simulink model "zynqRadioHWSWQPSKAD9361AD9364SL"  (R2025a)
settings: Solver=FixedStepDiscrete  StartTime=0.0  StopTime=0.5  RelTol=1e-3
PreLoadFcn:
  | setTxBurstLength = 10000;
  | txtmsg = ['Zynq radio HW/SW Co-design ÞÞÞÞ']; % Use only printable characters
  | 
  | %------------------------------------------------------------------------------------------------------
  | if ~isequal(size(txtmsg),[1 31])
  |     error('txtmsg must contain 31 characters');
  | end
  | 
  | [dataBits,msg] = zynqRadioHWSWQPSKgenHelloworldMsg(20); % generate 20 msgs for LUT
  | msgLUT = uint8(msg);
  | dataBitsLUT = dataBits(:);
  | Rsym                = 10e3;%1.92e6;
  | Config = zynqRadioHWSWQPSKTxRxParameters;
  | fs = Rsym*Config.SamplesPerSymbol;
  | word = [txtmsg newline];  % append a new line character to txtmsg
  | 
  | % The highest clock rate is 16 times the message character rate.
  | % As the message characters are fed at highest clock to FPGA
  | % repeat each character 16 times to maintain the message rate.
  | word = repelem(word.',16,1);
  | repeatTimes = ceil(setTxBurstLength/length(word));
  | inpData = complex(repmat(uint8(word),repeatTimes,1));
  | inUseTxBurstLength = length(inpData);
PostLoadFcn:
  | hScopeConfig = get_param([gcs '/HDL_QPSK/QPSK Tx Channel QPSK Rx/QPSK Rx/Frequency and Time Synchronizer/Symbol Synchronizer/No HDL/QPSK Receiver Eye Diagram'],'ScopeConfiguration');
  | hScopeConfig.OpenAtSimulationStart = false;
  | hScopeConfig.Visible = false;
  | clear hScopeConfig
InitFcn:
  | setTxBurstLength = 10000;
  | txtmsg = ['Zynq radio HW/SW Co-design ÞÞÞÞ']; % Use only printable characters
  | 
  | %------------------------------------------------------------------------------------------------------
  | if ~isequal(size(txtmsg),[1 31])
  |     error('txtmsg must contain 31 characters');
  | end
  | 
  | [dataBits,msg] = zynqRadioHWSWQPSKgenHelloworldMsg(20); % generate 20 msgs for LUT
  | msgLUT = uint8(msg);
  | dataBitsLUT = dataBits(:);
  | Rsym                = 10e3;%1.92e6;
  | Config = zynqRadioHWSWQPSKTxRxParameters;
  | fs = Rsym*Config.SamplesPerSymbol;
  | word = [txtmsg newline];  % append a new line character to txtmsg
  | 
  | % The highest clock rate is 16 times the message character rate.
  | % As the message characters are fed at highest clock to FPGA
  | % repeat each character 16 times to maintain the message rate.
  | word = repelem(word.',16,1);
  | repeatTimes = ceil(setTxBurstLength/length(word));
  | inpData = complex(repmat(uint8(word),repeatTimes,1));
  | inUseTxBurstLength = length(inpData);
  | 
  | Config.Preamble = logical(zeros(0,1))
undefined symbols (not defined in the file or in its folder): Add, dspblkCoreblockFVToolHelper, gcbh, gse_genframes, Shift
libraries: hdlsllib x144, simulink x37, dsphdlsigops2 x3, dsphdlfiltering2 x3, whdlutilities x3, dsphdlxfrm2 x2, dsphdlmathfun2 x2, commdigbbndpm3 x2, sdrzblksprivate x1
(part 6 of 6)

== matlab function zynqRadioHWSWQPSKAD9361AD9364SL/HDL_QPSK/QPSK Tx Channel QPSK Rx/QPSK Tx/FEC Encoder/DVB-S2 LDPC Encoder/ParityController ==
  data: ird_addr output; pwr_addr output; pwr_enb output; prd_addr output; endEnc input; paraddr input; encenable input; inpLen input; parLen input; qfactor input; noofcol input; reset input; starto output; endo output; valido output; par_ind output; i_index output; p_index output; framevalid input
function [ird_addr,pwr_addr,pwr_enb,prd_addr,starto,endo,valido,par_ind,...
    i_index,p_index] = ParityController(endEnc,paraddr,encenable,...
    inpLen,parLen,qfactor,noofcol,reset,framevalid)

persistent validO prdAddr pwrAddr pwrEnb pwrEnbReg ...
    irdAddr prdEnb endValid startO icountZ inCount ...
    parCount pcountZ outCount;
if isempty(validO)
    validO = false;
    prdAddr = uint8(1);
    pwrAddr = uint8(0);
    irdAddr = uint8(1);
    pwrEnb = false;
    pwrEnbReg = false;
    prdEnb = false;
    endValid = false;
    startO = false;
    icountZ = fi(1,0,9,0,hdlfimath);
    pcountZ = fi(1,0,9,0,hdlfimath);
    inCount = fi(0,0,16,0,hdlfimath);
    parCount = fi(0,0,16,0,hdlfimath);
    outCount = fi(0,0,16,0,hdlfimath);
end

ird_addr = irdAddr;
pwr_addr = pwrAddr;
prd_addr = prdAddr;
pwr_enb =  pwrEnbReg;
starto = startO;
par_ind = prdEnb;

i_index = icountZ;
p_index = pcountZ;

% Control signals
startO = endEnc;
endo = endValid;
valido = validO;

pwrEnbReg(:) = pwrEnb;

if reset
    prdAddr(:) = 1;
    pwrAddr(:) = 0;
    pwrEnb(:) = false;
    prdEnb(:) = false;
    irdAddr(:) = 1;
    icountZ(:) = 1;
    pcountZ(:) = 1;
    inCount(:) = 0;
    parCount(:) = 0;
else
    if validO
        pwrEnb(:) = false;
        pwrAddr(:) = 0;

        if ~prdEnb
            if icountZ == fi(360,0,9,0,hdlfimath)
                if ~(irdAddr == noofcol)
                    irdAddr(:) = irdAddr + 1;
                end
                icountZ(:) = 1;
            else
                icountZ(:) = icountZ + 1;
            end
        end

        if inCount == inpLen
            prdEnb(:) = true;
        else
            inCount(:) = inCount + 1;
        end

        if prdEnb
            if parCount == parLen
                prdEnb(:) = false;
            else
                parCount(:) = parCount + 1;
                if prdAddr == fi(qfactor,0,9,0,hdlfimath)
                    prdAddr(:) = 1;
                    if pcountZ == fi(360,0,9,0,hdlfimath)
                        pcountZ(:) = 1;
                    else
                        pcountZ(:) = pcountZ + 1;
                    end
                else
                    prdAddr(:) = prdAddr + 1;
                end
            end
        else
            prdAddr(:) = 1;
        end
    else
        if framevalid
            pwrEnb(:) = true;
            if pwrAddr == uint8(255)
                pwrAddr(:) = 1;
            else
                pwrAddr(:) = pwrAddr+1;
            end
        else
            if encenable
                pwrEnb(:) = true;
            else
                pwrEnb(:) = false;
            end
            pwrAddr(:) = prdAddr;
        end
        prdAddr(:) = paraddr;
        prdEnb(:) = false;
    end
end

if reset
    validO(:) = false;
    outCount(:) = 0;
elseif endEnc
    validO(:) = true;
    outCount(:) = 1;
else
    if validO
        if outCount == inpLen + parLen
            endValid(:) = true;
            outCount(:) = 0;
            validO(:) = false;
        else
            endValid(:) = false;
            outCount(:) = outCount+1;
        end
    else
        validO(:) = false;
        endValid(:) = false;
    end
end

== matlab function zynqRadioHWSWQPSKAD9361AD9364SL/HDL_QPSK/QPSK Tx Channel QPSK Rx/QPSK Tx/FEC Encoder/DVB-S2 LDPC Encoder/inputController ==
  data: reset output; datai input; iwr_data output size=360; iwr_addr output; starti input; endi input; validi input; fecframe input; coderate input; iwr_enb output size=1; ird_addr output; encenable output; addridx output; rdenable input; encend input; framevalid output; noofcol input
function [reset,iwr_data, iwr_addr,iwr_enb,ird_addr,encenable,addridx,framevalid] = ...
    inputController(datai,starti,endi,validi,fecframe,coderate,rdenable,encend,noofcol)
%#codegen

persistent fecFrame codeRate dataReg endReg validReg frameValid  frameValidReg...
           iwrData iwrAddr iwrEnb irdAddr idxCount wrCount encEnb disValid;
if isempty(dataReg)
    fecFrame = fi(0,0,1,0);
    codeRate = fi(0,0,4,0);
    dataReg = cast(0,'like',datai);
    endReg = false;
    validReg = false;
    frameValid = false;
    frameValidReg = false;
    iwrData = cast(zeros(360,1),'like',datai);
    iwrAddr = fi(0,0,8,0,hdlfimath);
    iwrEnb  = zeros(1,1)>0;
    irdAddr = fi(0,0,8,0,hdlfimath);
    idxCount = fi(1,0,9,0,hdlfimath);
    wrCount = fi(1,0,8,0,hdlfimath);
    encEnb = false;
    disValid = false;
end

% outputs
iwr_data = iwrData;
iwr_addr = iwrAddr;
iwr_enb = iwrEnb;
ird_addr = irdAddr;
encenable = disValid;

%% reset signal
reset = starti && validi;

%% Sample fecFrame and codeRate - Calculate input,parity length and address index.
if reset
    fecFrame(:) = fecframe;
    codeRate(:) = coderate;
end

addridx = fi(bitconcat(fecFrame,codeRate),0,5,0);

%% Reading data
if reset
    irdAddr(:) = 1;
else
    if rdenable
        if irdAddr == cast(noofcol,'like',irdAddr)
            irdAddr(:) = 1;
        else
            irdAddr(:) = irdAddr + 1;
        end
    end
end

%% Writing and Reading data into Input Bits RAM
if reset
    iwrData(:) = zeros(360,1);
    iwrAddr(:) = 0;
    iwrEnb(:) = zeros(1,1);
    idxCount(:) = 1;
    wrCount(:) = 1;
else
    if frameValid && validReg
         iwrEnb = true;
        for idx = 1:360
            if idxCount == fi(idx,0,9,0)
                iwrData(idx) = dataReg;
            end
        end
        iwrAddr(:) = wrCount;
        if idxCount == fi(360,0,9,0)
            idxCount(:) = 1;
            wrCount(:) = wrCount + 1;
        else
            idxCount(:) = idxCount + 1;
        end
    else
        % iwrData(:) = 0;
        iwrEnb(:)  = false;
    end
end

if reset
    frameValid(:) = true;
    encEnb(:) = false;
elseif endReg && validReg
    frameValid(:) = false;
    encEnb(:) = true;
elseif encend
    encEnb(:) = false;
end

if reset
    frameValidReg(:) = true;
elseif endi && validi
    frameValidReg(:) = false;
end

if encEnb
    disValid(:) = ~disValid;
else
    disValid(:) = false;
end

framevalid = frameValidReg;

dataReg(:) = datai;
endReg(:) = endi;
validReg(:) = validi;

== matlab function zynqRadioHWSWQPSKAD9361AD9364SL/HDL_QPSK/QPSK Tx Channel QPSK Rx/QPSK Rx/Frequency and Time Synchronizer/Packet Controller/MATLAB Function ==
  data: valid input; syncPulse input; out output
function out = fcn(valid,syncPulse)
%#codegen

  persistent Reg;
  if isempty(Reg)
      Reg = false;
  end
  
  out = Reg;
  
  if Reg && valid
      Reg = false;
  end
  
  if syncPulse
      Reg = true;
  end
  
end

== matlab function zynqRadioHWSWQPSKAD9361AD9364SL/HDL_QPSK/QPSK Tx Channel QPSK Rx/QPSK Rx/Frequency and Time Synchronizer/Symbol Synchronizer/Rate Handle/FIFO/Validate Input Push Pop/MATLAB Function ==
  data: rst input; count output; enb input; dir input; initVal parameter; countToVal parameter
function count = hdlCounter(rst,enb,dir,initVal,countToVal)
%#codegen

persistent countReg

if(isempty(countReg))
    countReg = fi(initVal,0,nextpow2(countToVal+1),0);
end

if(rst)
    countReg(:) = initVal;
elseif(enb)
    if(dir)
        if(countReg==countToVal)
            countReg(:) = initVal;
        else
            countReg(:) = countReg+1;
        end
    else
        if(countReg==initVal)
            countReg(:) = countToVal;
        else
            countReg(:) = countReg-1;
        end
    end
end

count = countReg;

end

== matlab function zynqRadioHWSWQPSKAD9361AD9364SL/HDL_QPSK/QPSK Tx Channel QPSK Rx/QPSK Tx/Bit Packetizer/Data Bits FIFO/MATLAB Function1 ==
  data: wr input; full output; rd input; dataBitsPerPacket parameter
function full = fcn(wr,rd,dataBitsPerPacket)
%#codegen
     
    depth = dataBitsPerPacket*2 - 1;
    persistent count;
    if isempty(count)
        count = fi(0,0,nextpow2(depth),0,hdlfimath);
    end

    if wr
        count(:) = count + 1;
    end
    if rd
        count(:) = count - 1;
    end

    full = (count > depth);

end

== matlab function zynqRadioHWSWQPSKAD9361AD9364SL/HDL_QPSK/QPSK Tx Channel QPSK Rx/QPSK Rx/Frequency and Time Synchronizer/Packet Controller/sample discard controller ==
  data: dataIn input; validIn input; dataOut output; startIn input; endIn input; startOut output; endOut output; validOut output
function [dataOut,startOut,endOut,validOut] = controller(dataIn,validIn,startIn,endIn)
%#codegen

   persistent active dataOutReg validOutReg startOutReg endOutReg;
   if isempty(active)
      active  = false;
      dataOutReg = cast(0,'like',dataIn);
      validOutReg = false;
      startOutReg = false;
      endOutReg = false;
   end
   
   dataOut = dataOutReg;
   validOut = validOutReg;
   startOut = startOutReg;
   endOut = endOutReg;
   
   startOutReg = startIn;
   endOutReg = endIn;
   
   if startIn
       active = true;
   end
   
   if active
       dataOutReg(:) = dataIn;
       validOutReg = validIn;
   else
       dataOutReg(:) = 0;
       validOutReg = false;
   end
   
   if endIn
       if active 
           endOutReg = true;
       else
           endOutReg = false;
       end
       active = false;
   end
end

== matlab function zynqRadioHWSWQPSKAD9361AD9364SL/HDL_QPSK/QPSK Tx Channel QPSK Rx/QPSK Rx/Frequency and Time Synchronizer/Symbol Synchronizer/Interpolation Control ==
  data: mu output; Delta input; Underflow output
function [mu,Underflow] = Interpolation_ctrl(Delta)
% Implementation of modulo-1 counter for interpolation control listed in
% Figure 8.4.19 of "Digital Communications - A Discrete-Time Approach"
% by Michael Rice. See design details in Chapter 8.4.3 of the same book.
% 
% Input:
%   Delta - Loop filter output. If loop is in lock, delta would be small
% Output:
%   Underflow - Indicator of counter underflow. This is the strobe signal
%               for downstream processing
%   mu - Difference between actual sampling instant and the optimal instant,
%        between zero and one
%#codegen

% countReg - Counter value delayed by 1 sample
% muReg - The estimated timing error normalized by half QPSK symbols

   mask = fi(1-2^(-10),1,11,10);
   
   persistent countReg underflowReg muReg;
   if isempty(countReg)
       countReg  = fi(0,1,11,10);
       muReg = fi(0,1,11,10);
       underflowReg = false;
   end
   
   
   Underflow = underflowReg;
   mu = muReg;   
   
   
   counter = bitand(mask,countReg)-Delta-fi(0.25,1,11,10); % decrementing counter
   
   % if countReg is a nonnegative number,
   % then mod(countReg,1) equals the fractional part of countReg
   if counter < 0
       underflowReg = true;
       muReg = bitshift(bitand(mask,countReg),2);
       countReg = fi(counter+1,1,11,10);% create underflow to counter
   else
       underflowReg = false;
       countReg = fi(counter,1,11,10);
   end
   


end

== matlab function zynqRadioHWSWQPSKAD9361AD9364SL/HDL_QPSK/QPSK Tx Channel QPSK Rx/QPSK Rx/Frequency and Time Synchronizer/Preamble Detector/Correlator/ThresholdLimiter ==
  settings: fimath=hdlfimath
  data: x input; y output
function y = applyLowerLimit(x)
    % Apply a lower limit to the threshold.
    %#codegen
    
    % Threshold is computed by summing across 63 samples.
    % Set lower limit to be equivalent of all 63 samples
    % having their LSB set to 1 and all others set to 0. 
    lowerLimit = cast(0.01, 'like', x);
    
    if x < lowerLimit
        y = lowerLimit;
    else
        y = x;
    end
end

== matlab function zynqRadioHWSWQPSKAD9361AD9364SL/Mock FRFT/Subsystem/frft_peaksearch ==
  data: sigIn input size=4000; sigOut output size=4000; validIn input size=1; validOut output size=1; p_max output; n_iterations parameter; p_low parameter; p_high parameter
function [sigOut, validOut, p_max] = frft_peaksearch( ...
                                            sigIn, validIn, ... % Ports
                                            n_iterations, p_low, p_high)... % Params
%#codegen
%FRFT_TRANSFORM Peak search in FRFT domain
%   1D Maximum peak search to identify optimum FRFT power

% If no valid input, only output 0.
if (~validIn)
    validOut = false;
    sigOut = double(zeros(size(sigIn)));
    p_max = double(0);

% ValidIn
else
    sig_reg = complex(double(sigIn));

    % Do Peak Search:
    [p_opt, ~] = find_frft_peak(sig_reg,n_iterations, [p_low,p_high], false);
    p_max = double(p_opt);

    sigOut = frft(sig_reg, p_max);
    validOut = true;

end




end
% END frft_transform
